simulink model "controller"  (R2023b)
settings: Solver=FixedStepAuto  StartTime=0.0  StopTime=10.0  FixedStep=1/100  RelTol=1e-3
undefined symbols (not defined in the file): MAX_TORQUE, MAX_TORQUE_REVERSE
libraries: simulink x7
settings Model: Creator=DAUIN-Win10  LastModifiedBy=Matteo
settings OptimizationCC: ReuseModelBlockBuffer=off
settings DebuggingCC: UnconnectedInputMsg=warning  UnconnectedOutputMsg=warning  UnconnectedLineMsg=warning
settings ModelReferenceCC: EnableRefExpFcnMdlSchedulingChecks=on
settings RTWCC: DLArmComputeVersion=19.05

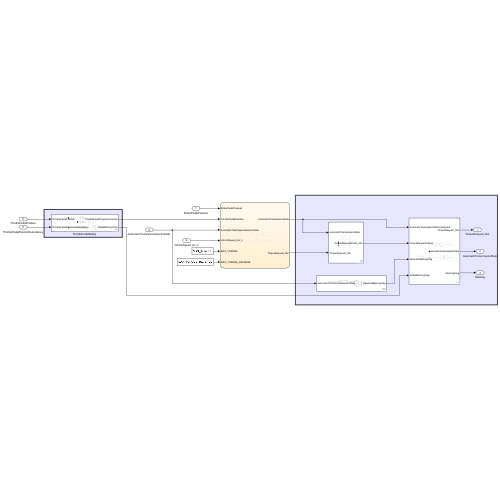
[thumbnail: Simulink's stored preview of the top-level diagram]
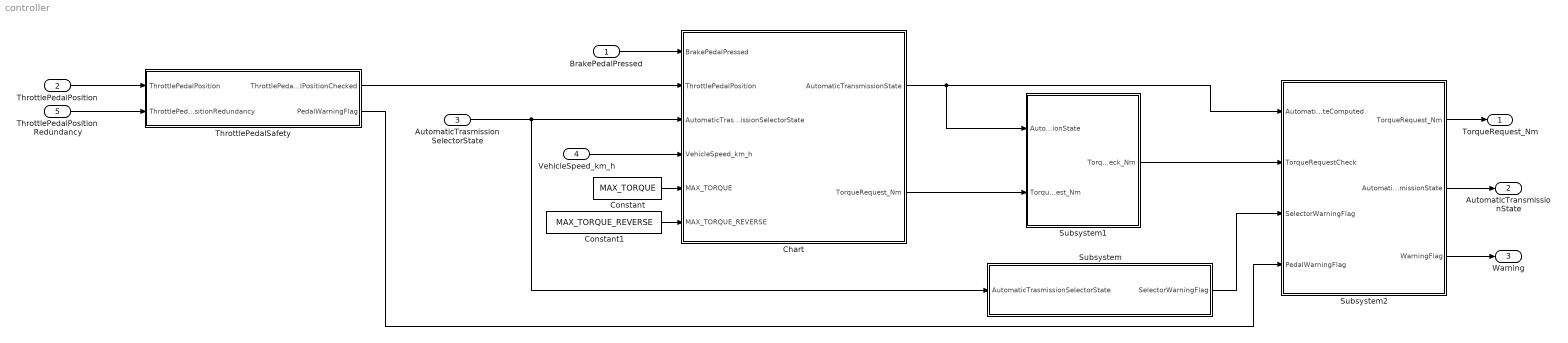
== system controller ==
  BrakePedalPressed : Inport  OutDataTypeStr=boolean
  ThrottlePedalPosition : Inport  Port=2  OutDataTypeStr=single
  AutomaticTrasmissionSelectorState : Inport  Port=3  OutDataTypeStr=Enum: TransmissionState
  VehicleSpeed_km_h : Inport  Port=4  OutDataTypeStr=single  Unit=km/h
  ThrottlePedalPositionRedundancy : Inport  Port=5  OutDataTypeStr=single
  Chart : Stateflow chart  TreatAsAtomicUnit=on
  Constant : Constant  Value=MAX_TORQUE
  Constant1 : Constant  Value=MAX_TORQUE_REVERSE
  Subsystem : Subsystem
  Subsystem1 : Subsystem
  Subsystem2 : Subsystem
  "ThrottlePedalSafety " : Subsystem
  TorqueRequest_Nm : Outport  OutDataTypeStr=single  Unit=N*m
  AutomaticTransmissionState : Outport  Port=2  OutDataTypeStr=Enum: TransmissionState
  Warning : Outport  Port=3
  wires:
  AutomaticTrasmissionSelectorState/1 -> Subsystem/1(AutomaticTrasmissionSelectorState), Chart/3(AutomaticTrasmissionSelectorState)
  Chart/1(AutomaticTransmissionState) -> Subsystem2/1(AutomaticTrasmissionStateComputed), Subsystem1/1(AutomaticTransmissionState)
  BrakePedalPressed/1 -> Chart/1(BrakePedalPressed)
  Constant/1 -> Chart/5(MAX_TORQUE)
  VehicleSpeed_km_h/1 -> Chart/4(VehicleSpeed_km_h)
  "ThrottlePedalSafety "/1(ThrottlePedalPositionChecked) -> Chart/2(ThrottlePedalPosition)
  Constant1/1 -> Chart/6(MAX_TORQUE_REVERSE)
  ThrottlePedalPosition/1 -> "ThrottlePedalSafety "/1(ThrottlePedalPosition)
  ThrottlePedalPositionRedundancy/1 -> "ThrottlePedalSafety "/2(ThrottlePedalPositionRedundancy)
  Chart/2(TorqueRequest_Nm) -> Subsystem1/2(TorqueRequest_Nm)
  Subsystem1/1(TorqueRequestCheck_Nm) -> Subsystem2/2(TorqueRequestCheck)
  Subsystem/1(SelectorWarningFlag) -> Subsystem2/3(SelectorWarningFlag)
  "ThrottlePedalSafety "/2(PedalWarningFlag) -> Subsystem2/4(PedalWarningFlag)
  Subsystem2/3(WarningFlag) -> Warning/1
  Subsystem2/2(AutomaticTransmissionState) -> AutomaticTransmissionState/1
  Subsystem2/1(TorqueRequest_Nm) -> TorqueRequest_Nm/1

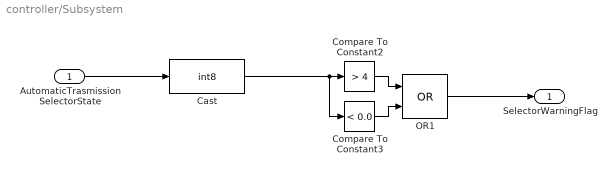
== system controller/Subsystem ==
  AutomaticTrasmissionSelectorState : Inport
  Cast : DataTypeConversion  OutDataTypeStr=int8  SaturateOnIntegerOverflow=off  RndMeth=Floor
  Compare To Constant2 : simulink/Logic and Bit Operations/Compare To Constant  relop=>  const=4  OutDataTypeStr=boolean
  Compare To Constant3 : simulink/Logic and Bit Operations/Compare To Constant  relop=<  const=0.0  OutDataTypeStr=boolean
  OR1 : Logic  Operator=OR  IconShape=distinctive  AllPortsSameDT=off  OutDataTypeStr=boolean
  SelectorWarningFlag : Outport
  wires:
  AutomaticTrasmissionSelectorState/1 -> Cast/1
  OR1/1 -> SelectorWarningFlag/1
  Cast/1 -> Compare To Constant3/1, Compare To Constant2/1
  Compare To Constant2/1 -> OR1/1
  Compare To Constant3/1 -> OR1/2

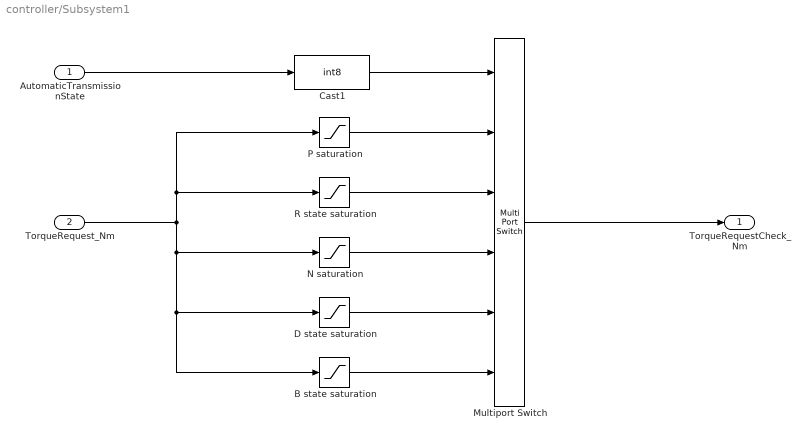
== system controller/Subsystem1 ==
  AutomaticTransmissionState : Inport
  TorqueRequest_Nm : Inport  Port=2
  B state saturation : Saturate  UpperLimit=MAX_TORQUE  LowerLimit=-MAX_TORQUE
  Cast1 : DataTypeConversion  OutDataTypeStr=int8  SaturateOnIntegerOverflow=off  RndMeth=Floor
  D state saturation : Saturate  UpperLimit=MAX_TORQUE  LowerLimit=0
  Multiport Switch : MultiPortSwitch  DataPortOrder=Specify indices  Inputs=5  DataPortIndices={0,1,2,3,4}  SaturateOnIntegerOverflow=off  InputSameDT=off
  N saturation : Saturate  UpperLimit=0  LowerLimit=0
  P saturation : Saturate  UpperLimit=0  LowerLimit=0
  R state saturation : Saturate  UpperLimit=0  LowerLimit=-MAX_TORQUE_REVERSE
  TorqueRequestCheck_Nm : Outport
  wires:
  B state saturation/1 -> Multiport Switch/6
  TorqueRequest_Nm/1 -> R state saturation/1, P saturation/1, D state saturation/1, B state saturation/1, N saturation/1
  N saturation/1 -> Multiport Switch/4
  R state saturation/1 -> Multiport Switch/3
  P saturation/1 -> Multiport Switch/2
  Multiport Switch/1 -> TorqueRequestCheck_Nm/1
  Cast1/1 -> Multiport Switch/1
  D state saturation/1 -> Multiport Switch/5
  AutomaticTransmissionState/1 -> Cast1/1

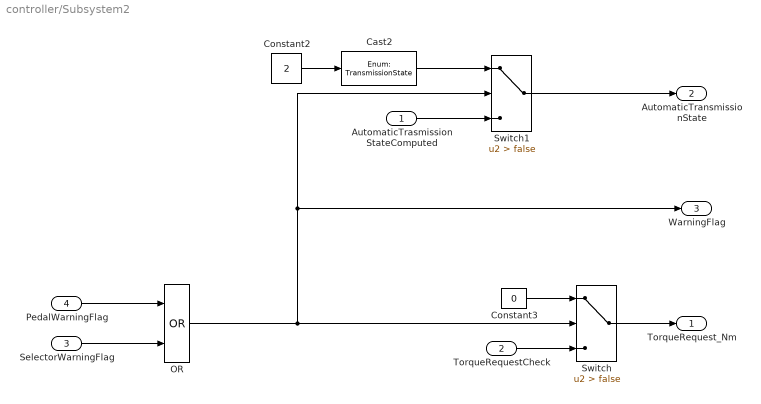
== system controller/Subsystem2 ==
  AutomaticTrasmissionStateComputed : Inport
  TorqueRequestCheck : Inport  Port=2
  SelectorWarningFlag : Inport  Port=3
  PedalWarningFlag : Inport  Port=4
  Cast2 : DataTypeConversion  OutDataTypeStr=Enum: TransmissionState  SaturateOnIntegerOverflow=off  RndMeth=Floor
  Constant2 : Constant  Value=2  OutDataTypeStr=int8
  Constant3 : Constant  Value=0
  OR : Logic  Operator=OR  IconShape=distinctive  AllPortsSameDT=off  OutDataTypeStr=boolean
  Switch : Switch  Criteria=u2 > Threshold  Threshold=false  SaturateOnIntegerOverflow=off  InputSameDT=off
  Switch1 : Switch  Criteria=u2 > Threshold  Threshold=false  SaturateOnIntegerOverflow=off  InputSameDT=off
  TorqueRequest_Nm : Outport  OutDataTypeStr=single  Unit=N*m
  AutomaticTransmissionState : Outport  Port=2  OutDataTypeStr=Enum: TransmissionState
  WarningFlag : Outport  Port=3  OutDataTypeStr=boolean
  wires:
  Cast2/1 -> Switch1/1
  Constant3/1 -> Switch/1
  OR/1 -> Switch/2, WarningFlag/1, Switch1/2
  Switch/1 -> TorqueRequest_Nm/1
  Constant2/1 -> Cast2/1
  Switch1/1 -> AutomaticTransmissionState/1
  AutomaticTrasmissionStateComputed/1 -> Switch1/3
  TorqueRequestCheck/1 -> Switch/3
  PedalWarningFlag/1 -> OR/1
  SelectorWarningFlag/1 -> OR/2

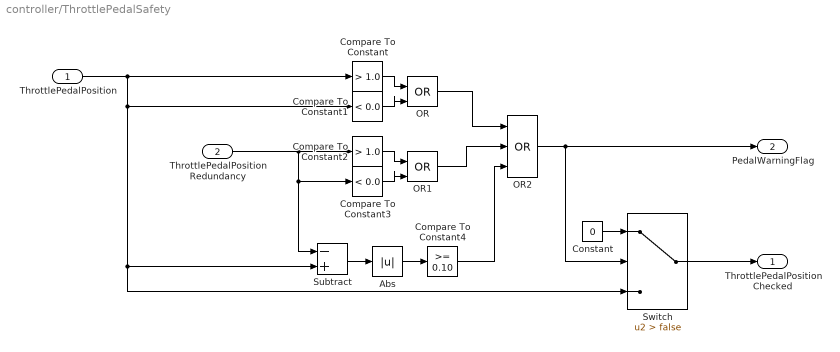
== system controller/ThrottlePedalSafety  ==
  ThrottlePedalPosition : Inport  OutDataTypeStr=single
  ThrottlePedalPositionRedundancy : Inport  Port=2  OutDataTypeStr=single
  Abs : Abs  SaturateOnIntegerOverflow=off
  Compare To Constant : simulink/Logic and Bit Operations/Compare To Constant  relop=>  const=1.0  OutDataTypeStr=boolean
  Compare To Constant1 : simulink/Logic and Bit Operations/Compare To Constant  relop=<  const=0.0  OutDataTypeStr=boolean
  Compare To Constant2 : simulink/Logic and Bit Operations/Compare To Constant  relop=>  const=1.0  OutDataTypeStr=boolean
  Compare To Constant3 : simulink/Logic and Bit Operations/Compare To Constant  relop=<  const=0.0  OutDataTypeStr=boolean
  Compare To Constant4 : simulink/Logic and Bit Operations/Compare To Constant  relop=>=  const=0.10  OutDataTypeStr=boolean
  Constant : Constant  Value=0  OutDataTypeStr=single
  OR : Logic  Operator=OR  IconShape=distinctive  AllPortsSameDT=off  OutDataTypeStr=boolean
  OR1 : Logic  Operator=OR  IconShape=distinctive  AllPortsSameDT=off  OutDataTypeStr=boolean
  OR2 : Logic  Operator=OR  Inputs=3  IconShape=distinctive  AllPortsSameDT=off  OutDataTypeStr=boolean
  Subtract : Sum  Inputs=-+
  Switch : Switch  Criteria=u2 > Threshold  Threshold=false  SaturateOnIntegerOverflow=off  InputSameDT=off
  ThrottlePedalPositionChecked : Outport  OutDataTypeStr=single
  PedalWarningFlag : Outport  Port=2  OutDataTypeStr=boolean
  wires:
  ThrottlePedalPosition/1 -> Compare To Constant/1, Compare To Constant1/1, Subtract/2, Switch/3
  Subtract/1 -> Abs/1
  Abs/1 -> Compare To Constant4/1
  Constant/1 -> Switch/1
  Switch/1 -> ThrottlePedalPositionChecked/1
  OR2/1 -> PedalWarningFlag/1, Switch/2
  Compare To Constant1/1 -> OR/2
  Compare To Constant/1 -> OR/1
  Compare To Constant2/1 -> OR1/1
  Compare To Constant3/1 -> OR1/2
  ThrottlePedalPositionRedundancy/1 -> Subtract/1, Compare To Constant3/1, Compare To Constant2/1
  Compare To Constant4/1 -> OR2/3
  OR1/1 -> OR2/2
  OR/1 -> OR2/1

== stateflow chart controller/Chart ==
  settings: executeAtInitialization=1
  state BRAKE
    state NOMINAL_BRAKE
      entry:
      AutomaticTransmissionState=TransmissionState.Brake;
      stopping=0;
      during:
      if(ThrottlePedalPosition > 1/3)
      TorqueRequest_Nm = MAX_TORQUE * (3/2) * (ThrottlePedalPosition-1/3);
      elseif (ThrottlePedalPosition<=1/3 && VehicleSpeed_km_h>0)
      TorqueRequest_Nm = -MAX_TORQUE * (1-3*ThrottlePedalPosition);
      elseif (ThrottlePedalPosition<=1/3 && VehicleSpeed_km_h<0)
      TorqueRequest_Nm=single(0);
      stopping = 1;
      end
    state STOPPING
      entry:
      Kp = 0.5; %h/Km
      during:
      if(VehicleSpeed_km_h<0)
      TorqueRequest_Nm=Kp*MAX_TORQUE*(-VehicleSpeed_km_h);
      else
      TorqueRequest_Nm=0;
      stopping=0;
      end
    (default) -> NOMINAL_BRAKE
    NOMINAL_BRAKE -> STOPPING : [stopping==1]
    STOPPING -> NOMINAL_BRAKE : [stopping==0]
  state PARK
    entry:
    AutomaticTransmissionState=TransmissionState.Park;
    during:
    TorqueRequest_Nm = single(0);
  state DRIVE
    entry:
    AutomaticTransmissionState=TransmissionState.Drive;
    during:
    TorqueRequest_Nm = MAX_TORQUE*ThrottlePedalPosition;
  state NEUTRAL
    entry:
    AutomaticTransmissionState=TransmissionState.Neutral;
    during:
    TorqueRequest_Nm = single(0);
  state REVERSE
    entry:
    AutomaticTransmissionState=TransmissionState.Reverse;
    during:
    TorqueRequest_Nm = -MAX_TORQUE_REVERSE*ThrottlePedalPosition;
  (default) -> PARK
  NEUTRAL -> PARK [order 3] : [abs(VehicleSpeed_km_h)<5 && BrakePedalPressed==1 ...
      |  && AutomaticTrasmissionSelectorState<TransmissionState.Reverse]
  PARK -> NEUTRAL : [BrakePedalPressed==1 ...
      | && AutomaticTrasmissionSelectorState>TransmissionState.Park]
  DRIVE -> BRAKE [order 1] : [ThrottlePedalPosition>1/3 ...
      | && AutomaticTrasmissionSelectorState>TransmissionState.Drive]
  BRAKE -> DRIVE : [AutomaticTrasmissionSelectorState<TransmissionState.Brake]
  DRIVE -> NEUTRAL [order 2] : [AutomaticTrasmissionSelectorState<TransmissionState.Drive]
  NEUTRAL -> REVERSE [order 2] : [VehicleSpeed_km_h<5 && BrakePedalPressed==1 ...
      | && (AutomaticTrasmissionSelectorState<TransmissionState.Neutral ...
      | && AutomaticTrasmissionSelectorState>TransmissionState.Park)]
  NEUTRAL -> DRIVE [order 1] : [VehicleSpeed_km_h>-5 && BrakePedalPressed==1 ...
      | && AutomaticTrasmissionSelectorState>TransmissionState.Neutral]
  REVERSE -> NEUTRAL : [AutomaticTrasmissionSelectorState>TransmissionState.Reverse]
  data: BrakePedalPressed input; ThrottlePedalPosition input; AutomaticTrasmissionSelectorState input; VehicleSpeed_km_h input; AutomaticTransmissionState output; TorqueRequest_Nm output; MAX_TORQUE input; MAX_TORQUE_REVERSE input; stopping local; Kp local
